simulink model "model"  (R2020b)
settings: Solver=VariableStepAuto  StartTime=0.0  StopTime=10.0  RelTol=1e-3
settings Model: Creator=Lenovo  LastModifiedBy=Lenovo

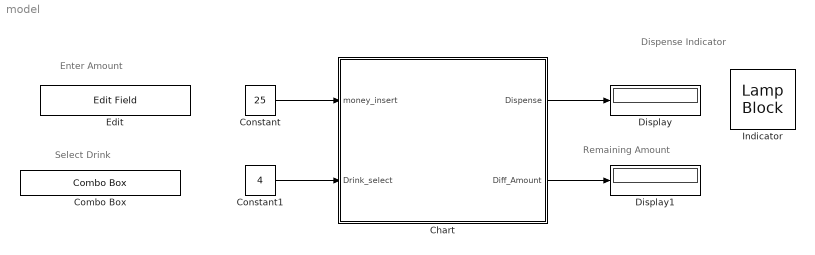
== system model ==
  note: Dispense Indicator
  note: Remaining Amount
  note: Select Drink
  note: Enter Amount
  Chart : Stateflow chart  TreatAsAtomicUnit=on
  Combo Box : ComboBox  LabelPosition=Hide  SelectedLabel=Sprite
      settings: Values={{'Coke', 'Pepsi', 'Soda', 'Sprite'}, [1 2 3 4]}
  Constant : Constant  Value=25
  Constant1 : Constant  Value=4
  Display : Display
  Display1 : Display
  Edit : EditField  LabelPosition=Hide  ShowInitialText=on  Alignment=Center
  Indicator : LampBlock
  wires:
  Constant/1 -> Chart/1(money_insert)
  Chart/1(Dispense) -> Display/1
  Constant1/1 -> Chart/2(Drink_select)
  Chart/2(Diff_Amount) -> Display1/1

== stateflow chart model/Chart ==
  state error
  state Coin_Inserted
  state Coke
  state Soda
  state Sprite
  state Pepsi
  (junction 23) -> error [order 2] : [money_insert<18]{Dispense=0}
  (default) -> Coin_Inserted
  Coin_Inserted -> error [order 1] : [money_insert<=0]{Dispense=0}
  Coin_Inserted -> (junction 23) [order 2] : [Drink_select==1]
  (junction 23) -> Coke [order 1] : [money_insert>=18]{Dispense=1, Diff_Amount=money_insert-18}
  (junction 28) -> error [order 2] : [money_insert<22]{Dispense=0}
  (junction 21) -> error [order 2] : [money_insert<20]{Dispense=0}
  (junction 16) -> error [order 2] : [money_insert<15]{Dispense=0}
  Coin_Inserted -> (junction 16) [order 4] : [Drink_select==3]
  Coin_Inserted -> (junction 21) [order 3] : [Drink_select==2]
  Coin_Inserted -> (junction 28) [order 5] : [Drink_select==4]
  (junction 16) -> Soda [order 1] : [money_insert>=15]{Dispense=1, Diff_Amount=money_insert-15}
  (junction 28) -> Sprite [order 1] : [money_insert>=22]{Dispense=1, Diff_Amount=money_insert-22}
  (junction 21) -> Pepsi [order 1] : [money_insert>=20]{Dispense=1, Diff_Amount=money_insert-20}
  data: money_insert input; Dispense output; Diff_Amount output; Drink_select input
